simulink model "Control_Simulation"  (R2015a)
settings: Solver=ode45  StartTime=0.0  StopTime=15000  MaxStep=1  RelTol=1e-3
InitFcn:
  | m = 1.33;
  | L = 0.1;
  | Jxx = m*L^2/12;
  | Jyy = m*L^2/12;
  | Jzz = m*L^2/12;
  | J = diag([Jxx, Jyy, Jzz]);
  | omega0 = [1 1 1];
  | 
  | phi0=0;
  | theta0=0;
  | psi0=0;
  | 
  | R0_ECIF_2_B = eye(3);
values from neighbouring files (symbols this model uses):
  Earth = wgs84Ellipsoid    [TrovaSorvoloConAngoli.m]    (also in calculate_orbit.m)
undefined symbols (not defined in the file or in its folder): WGS84
libraries: aerolibtransform2 x2, aerolib6dof2 x1, aerolibgravity2 x1
settings Model: Creator=mehdi  LastModifiedBy=mehdi

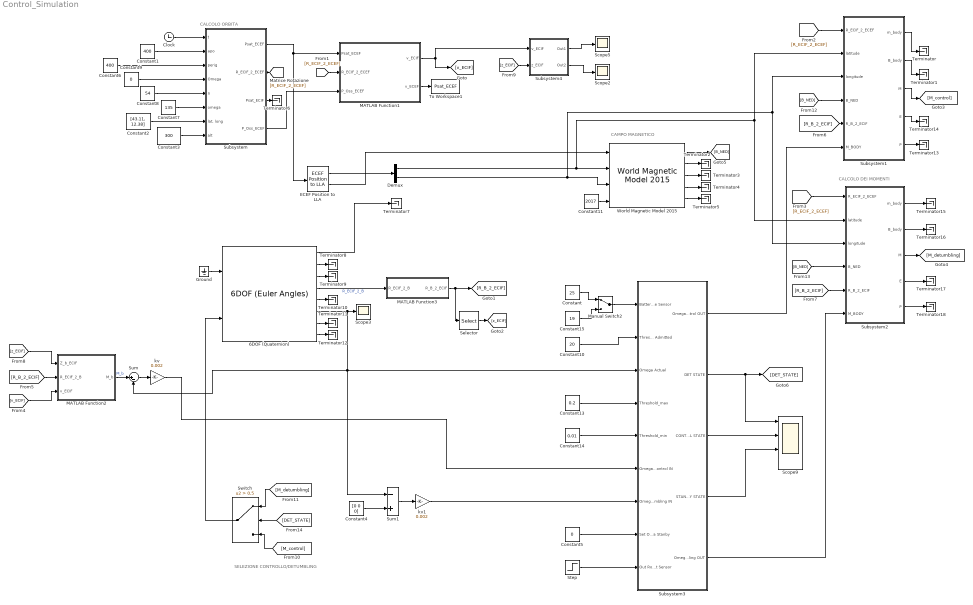
== system Control_Simulation ==
  note: SELEZIONE CONTROLLO/DETUMBLING
  note: CALCOLO DEI MOMENTI
  note: CAMPO MAGNETICO
  note: CALCOLO ORBITA
  6DOF (Quaternion) : aerolib6dof2/6DOF (Euler Angles)  units=Metric (MKS)  mtype=Fixed  rep=Quaternion  xme_0=[0 0 0]  Vm_0=[0 0 0]  eul_0=[0 0 0]  pm_0=omega0  mass_0=1.0  mass_e=0.5  mass_f=2.0  inertia=J  inertia_e=eye(3)  inertia_f=2*eye(3)  k_quat=1  vre_flag=on
  Clock : Clock
  Constant : Constant  Value=25
  Constant1 : Constant  Value=400
  Constant10 : Constant  Value=20
  Constant11 : Constant  Value=2017
  Constant13 : Constant  Value=0.2
  Constant14 : Constant  Value=0.01
  Constant15 : Constant  Value=19
  Constant2 : Constant  Value=[43.11, 12.38]
  Constant3 : Constant  Value=300
  Constant4 : Constant  Value=[0 0 0]
  Constant5 : Constant  Value=0
  Constant6 : Constant  Value=400
  Constant7 : Constant  Value=135
  Constant8 : Constant  Value=54
  Constant9 : Constant  Value=0
  Demux : Demux  Outputs=2
  ECEF Position to LLA : aerolibtransform2/ECEF Position to LLA  units=Metric (MKS)  ptype=Earth (WGS84)  F=1/298.257223563  R=6378137
  Ground : Ground
  MATLAB Function1 : MATLAB Function  TreatAsAtomicUnit=on
  MATLAB Function2 : MATLAB Function  TreatAsAtomicUnit=on
  MATLAB Function3 : MATLAB Function  TreatAsAtomicUnit=on
  Manual Switch2 : ManualSwitch
  Scope2 : Scope
      settings: YMin=0  YMax=14
  Scope3 : Scope
      settings: ShowLegends=on  YMin=-0.225  YMax=0.05  SaveName=v_ang
  Scope5 : Scope
      settings: YMin=-0.015  YMax=0.0175  SaveName=error_w
  Scope9 : Scope  NumInputPorts=4
      settings: TimeRange=1.404786680541292  YMin=-5~-5~-5~-5  YMax=5~5~5~5  SaveName=ScopeData8
  Selector : Selector  NumberOfDimensions=2  InputPortWidth=3  IndexOptions=Index vector (dialog),Index vector (dialog)  Indices=[1 2 3],3  OutputSizes=1,1
  Step : Step  SampleTime=0
  Subsystem : Subsystem
  Subsystem1 : Subsystem
  Subsystem2 : Subsystem
  Subsystem3 : Subsystem
  Subsystem4 : Subsystem
  Sum : Sum  Inputs=|+-
  Sum1 : Sum  Inputs=-+
  Switch : Switch  Criteria=u2 > Threshold  Threshold=0.5
  Terminator{,1..18} (19 alike) : Terminator
  To Workspace1 : ToWorkspace  VariableName=Psat_ECEF  SaveFormat=Structure With Time  SampleTime=-1
  World Magnetic Model 2015 : aerolibgravity2/World Magnetic Model 2015  units=Metric (MKS)  time_in=on  month=January  day=1  year=2015  action=Error  h_out=on  dec_out=on  inc_out=on  ti_out=on
  kv : Gain  Gain=0.002
  kv1 : Gain  Gain=0.002
  wires:
  MATLAB Function2/1(M_b) -> Sum/1  "M_b"
  6DOF (Quaternion)/4 -> MATLAB Function3/1(R_ECIF_2_B)  "R_ECIF_2_B"
  MATLAB Function3/1(R_B_2_ECIF) -> Selector/1, [R_B_2_ECIF]
  Sum/1 -> kv/1
  Clock/1 -> Subsystem/1(t)
  Constant1/1 -> Subsystem/2(apo)
  Constant6/1 -> Subsystem/3(perig)
  Constant9/1 -> Subsystem/4(Omega)
  Constant8/1 -> Subsystem/5(Ii)
  Constant7/1 -> Subsystem/6(omega)
  Constant2/1 -> Subsystem/7("lat, long")
  Constant3/1 -> Subsystem/8(alt)
  Subsystem/4(P_Oss_ECEF) -> MATLAB Function1/3(P_Oss_ECEF)
  Subsystem/1(Psat_ECEF) -> ECEF Position to LLA/1, MATLAB Function1/1(Psat_ECEF)
  ECEF Position to LLA/2 -> World Magnetic Model 2015/1
  Demux/1 -> World Magnetic Model 2015/2, Subsystem1/2(latitude), Subsystem2/2(latitude)
  Demux/2 -> Subsystem2/3(longitude), Subsystem1/3(longitude), World Magnetic Model 2015/3
  ECEF Position to LLA/1 -> Demux/1
  Subsystem1/2(B_body) -> Terminator1/1
  Constant11/1 -> World Magnetic Model 2015/4
  Subsystem1/1(m_body) -> Terminator/1
  MATLAB Function1/2(v_ECEF) -> To Workspace1/1
  World Magnetic Model 2015/2 -> Terminator2/1
  World Magnetic Model 2015/3 -> Terminator3/1
  World Magnetic Model 2015/4 -> Terminator4/1
  World Magnetic Model 2015/5 -> Terminator5/1
  Subsystem/3(Psat_ECIF) -> Terminator6/1
  6DOF (Quaternion)/1 -> Terminator7/1
  6DOF (Quaternion)/2 -> Terminator8/1
  6DOF (Quaternion)/3 -> Terminator9/1
  6DOF (Quaternion)/5 -> Terminator10/1
  6DOF (Quaternion)/7 -> Terminator11/1
  6DOF (Quaternion)/8 -> Terminator12/1
  Ground/1 -> 6DOF (Quaternion)/1
  6DOF (Quaternion)/6 -> Sum1/1, Subsystem3/3(Omega Actual), Sum/2, Scope3/1
  Constant4/1 -> Sum1/2
  Sum1/1 -> kv1/1
  Switch/1 -> 6DOF (Quaternion)/2
  Subsystem/2(R_ECIF_2_ECEF) -> [R_ECIF_2_ECEF]
  [R_ECIF_2_ECEF] -> MATLAB Function1/2(R_ECIF_2_ECEF)
  [R_ECIF_2_ECEF] -> Subsystem1/1(R_ECIF_2_ECEF)
  [R_ECIF_2_ECEF] -> Subsystem2/1(R_ECIF_2_ECEF)
  Constant10/1 -> Subsystem3/2(Threshold Admitted)
  Constant5/1 -> Subsystem3/8(Set Omega Stanby)
  Constant13/1 -> Subsystem3/4(Threshold_max)
  Constant14/1 -> Subsystem3/5(Threshold_min)
  Constant/1 -> Manual Switch2/1
  Constant15/1 -> Manual Switch2/2
  Manual Switch2/1 -> Subsystem3/1(Battery Charge Sensor)
  Subsystem3/2(DET STATE) -> [DET_STATE], Scope9/1
  Subsystem3/3(CONTROL STATE) -> Scope9/2
  Subsystem3/4(STANDBY STATE) -> Scope9/3
  Step/1 -> Subsystem3/9(Out Rocket Sensor)
  kv1/1 -> Subsystem3/7(Omega Dethumbling IN)
  kv/1 -> Subsystem3/6(Omega Control IN)
  Subsystem3/5(Omega Dethumbling OUT) -> Subsystem2/6(M_BODY)
  Subsystem3/1(Omega Control OUT) -> Subsystem1/6(M_BODY)
  Subsystem4/1(Out1) -> Scope5/1
  Subsystem4/2(Out2) -> Scope2/1
  Subsystem1/4(E) -> Terminator14/1
  Subsystem1/5("P ") -> Terminator13/1
  Subsystem2/1(m_body) -> Terminator15/1
  Subsystem2/2(B_body) -> Terminator16/1
  Subsystem2/4(E) -> Terminator17/1
  Subsystem2/5("P ") -> Terminator18/1
  MATLAB Function1/1(v_ECIF) -> Subsystem4/1(v_ECIF), [v_ECIF]
  [v_ECIF] -> MATLAB Function2/3(v_ECIF)
  [R_B_2_ECIF] -> MATLAB Function2/2(R_ECIF_2_B)
  [R_B_2_ECIF] -> Subsystem1/5(R_B_2_ECIF)
  [R_B_2_ECIF] -> Subsystem2/5(R_B_2_ECIF)
  Selector/1 -> [z_ECIF]
  [z_ECIF] -> MATLAB Function2/1(Z_b_ECIF)
  [z_ECIF] -> Subsystem4/2(z_ECIF)
  Subsystem1/3(M) -> [M_control]
  [M_control] -> Switch/3
  [M_detumbling] -> Switch/1
  Subsystem2/3(M) -> [M_detumbling]
  World Magnetic Model 2015/1 -> [B_NED]
  [B_NED] -> Subsystem1/4(B_NED)
  [B_NED] -> Subsystem2/4(B_NED)
  [DET_STATE] -> Switch/2

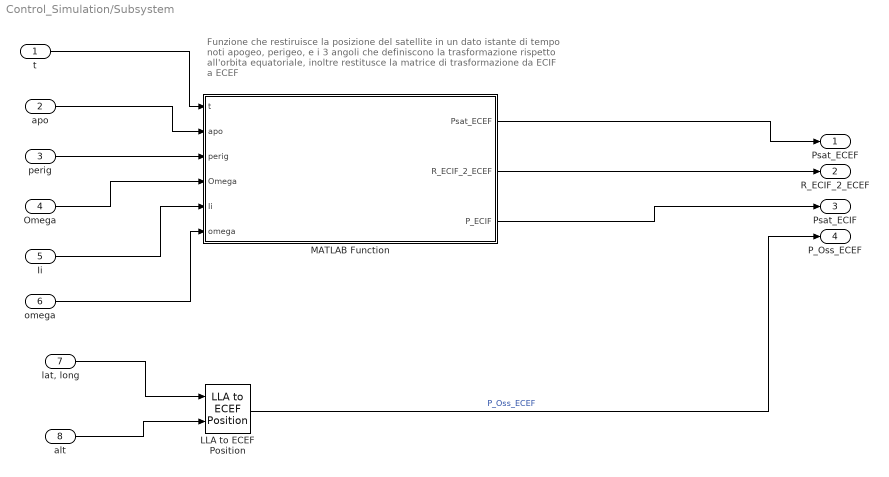
== system Control_Simulation/Subsystem ==
  note: Funzione che restiruisce la posizione del satellite in un dato
      | istante di tempo noti apogeo, perigeo, e i 3 angoli che definiscono
      | la trasformazione rispetto all'orbita equatoriale, inoltre
      | restitusce la matrice di trasformazione da ECIF a ECEF
  t : Inport
  apo : Inport  Port=2
  perig : Inport  Port=3
  Omega : Inport  Port=4
  Ii : Inport  Port=5
  omega : Inport  Port=6
  "lat, long" : Inport  Port=7
  alt : Inport  Port=8
  LLA to ECEF Position : aerolibtransform2/LLA to ECEF Position  units=Metric (MKS)  ptype=Earth (WGS84)  F=1/298.257223563  R=6378137
  MATLAB Function : MATLAB Function  TreatAsAtomicUnit=on
  Psat_ECEF : Outport
  R_ECIF_2_ECEF : Outport  Port=2
  Psat_ECIF : Outport  Port=3
  P_Oss_ECEF : Outport  Port=4
  wires:
  MATLAB Function/3(P_ECIF) -> Psat_ECIF/1
  t/1 -> MATLAB Function/1(t)
  apo/1 -> MATLAB Function/2(apo)
  perig/1 -> MATLAB Function/3(perig)
  omega/1 -> MATLAB Function/6(omega)
  Ii/1 -> MATLAB Function/5(Ii)
  Omega/1 -> MATLAB Function/4(Omega)
  alt/1 -> LLA to ECEF Position/2
  MATLAB Function/2(R_ECIF_2_ECEF) -> R_ECIF_2_ECEF/1
  LLA to ECEF Position/1 -> P_Oss_ECEF/1  "P_Oss_ECEF"
  "lat, long"/1 -> LLA to ECEF Position/1
  MATLAB Function/1(Psat_ECEF) -> Psat_ECEF/1

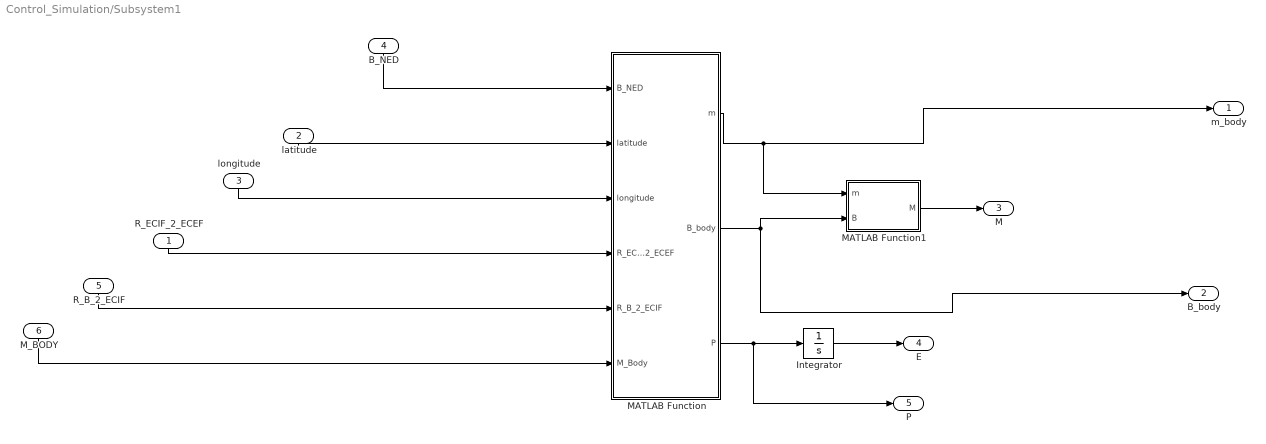
== system Control_Simulation/Subsystem1 ==
  R_ECIF_2_ECEF : Inport
  latitude : Inport  Port=2
  longitude : Inport  Port=3
  B_NED : Inport  Port=4
  R_B_2_ECIF : Inport  Port=5
  M_BODY : Inport  Port=6
  Integrator : Integrator
  MATLAB Function : MATLAB Function  TreatAsAtomicUnit=on
  MATLAB Function1 : MATLAB Function  TreatAsAtomicUnit=on
  m_body : Outport
  B_body : Outport  Port=2
  M : Outport  Port=3
  E : Outport  Port=4
  "P " : Outport  Port=5
  wires:
  B_NED/1 -> MATLAB Function/1(B_NED)
  R_B_2_ECIF/1 -> MATLAB Function/5(R_B_2_ECIF)
  longitude/1 -> MATLAB Function/3(longitude)
  R_ECIF_2_ECEF/1 -> MATLAB Function/4(R_ECIF_2_ECEF)
  latitude/1 -> MATLAB Function/2(latitude)
  MATLAB Function/1(m) -> MATLAB Function1/1(m), m_body/1
  M_BODY/1 -> MATLAB Function/6(M_Body)
  MATLAB Function/2(B_body) -> B_body/1, MATLAB Function1/2(B)
  MATLAB Function1/1(M) -> M/1
  MATLAB Function/3(P) -> "P "/1, Integrator/1
  Integrator/1 -> E/1

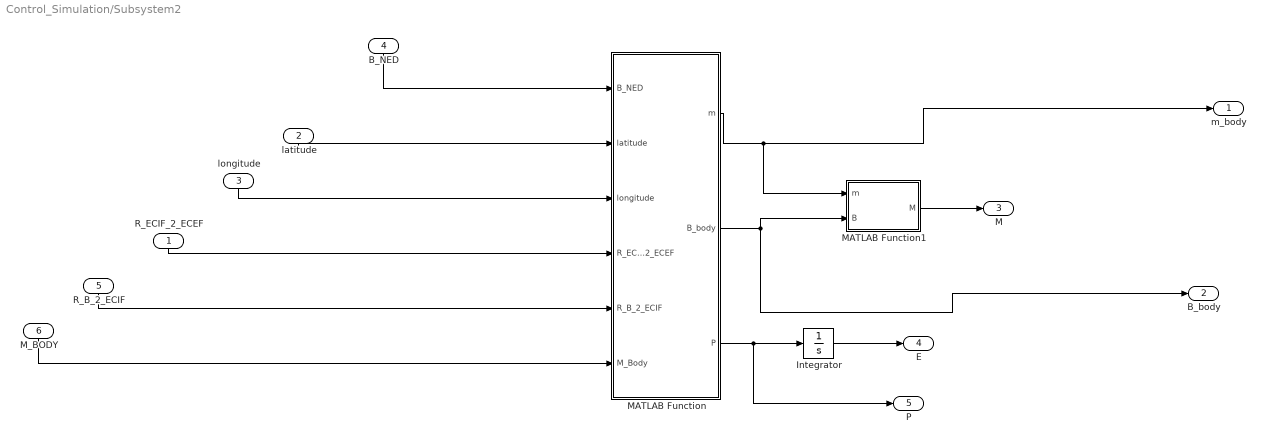
== system Control_Simulation/Subsystem2 ==
  R_ECIF_2_ECEF : Inport
  latitude : Inport  Port=2
  longitude : Inport  Port=3
  B_NED : Inport  Port=4
  R_B_2_ECIF : Inport  Port=5
  M_BODY : Inport  Port=6
  Integrator : Integrator
  MATLAB Function : MATLAB Function  TreatAsAtomicUnit=on
  MATLAB Function1 : MATLAB Function  TreatAsAtomicUnit=on
  m_body : Outport
  B_body : Outport  Port=2
  M : Outport  Port=3
  E : Outport  Port=4
  "P " : Outport  Port=5
  wires:
  B_NED/1 -> MATLAB Function/1(B_NED)
  R_B_2_ECIF/1 -> MATLAB Function/5(R_B_2_ECIF)
  longitude/1 -> MATLAB Function/3(longitude)
  R_ECIF_2_ECEF/1 -> MATLAB Function/4(R_ECIF_2_ECEF)
  latitude/1 -> MATLAB Function/2(latitude)
  MATLAB Function/1(m) -> MATLAB Function1/1(m), m_body/1
  M_BODY/1 -> MATLAB Function/6(M_Body)
  MATLAB Function/2(B_body) -> B_body/1, MATLAB Function1/2(B)
  MATLAB Function1/1(M) -> M/1
  MATLAB Function/3(P) -> "P "/1, Integrator/1
  Integrator/1 -> E/1

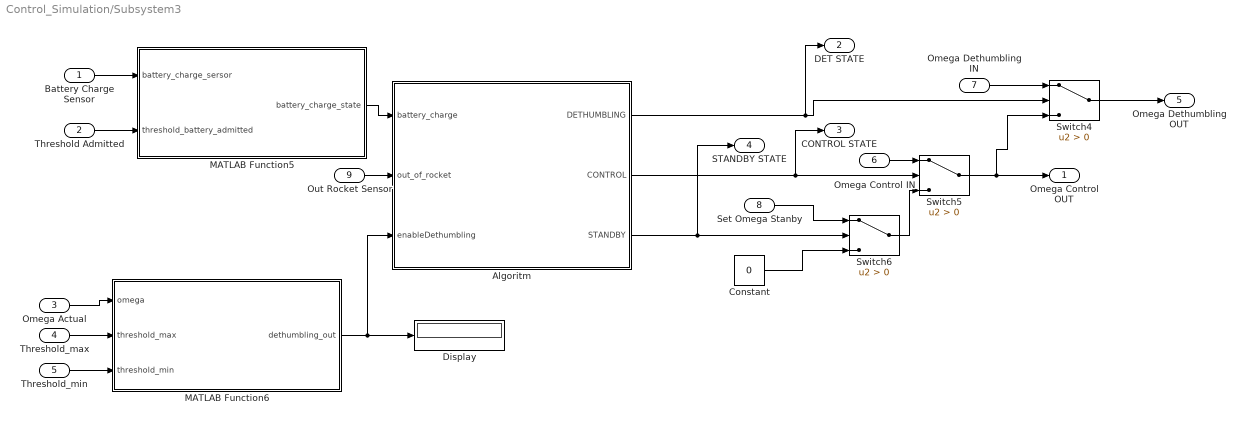
== system Control_Simulation/Subsystem3 ==
  Battery Charge Sensor : Inport
  Threshold Admitted : Inport  Port=2
  Omega Actual : Inport  Port=3
  Threshold_max : Inport  Port=4
  Threshold_min : Inport  Port=5
  Omega Control IN : Inport  Port=6
  Omega Dethumbling IN : Inport  Port=7
  Set Omega Stanby : Inport  Port=8
  Out Rocket Sensor : Inport  Port=9
  Algoritm : Stateflow chart  TreatAsAtomicUnit=on
  Constant : Constant  Value=0
  Display : Display
  MATLAB Function5 : MATLAB Function  TreatAsAtomicUnit=on
  MATLAB Function6 : MATLAB Function  TreatAsAtomicUnit=on
  Switch4 : Switch  Criteria=u2 > Threshold
  Switch5 : Switch  Criteria=u2 > Threshold
  Switch6 : Switch  Criteria=u2 > Threshold
  Omega Control OUT : Outport
  DET STATE : Outport  Port=2
  CONTROL STATE : Outport  Port=3
  STANDBY STATE : Outport  Port=4
  Omega Dethumbling OUT : Outport  Port=5
  wires:
  Threshold_max/1 -> MATLAB Function6/2(threshold_max)
  Omega Actual/1 -> MATLAB Function6/1(omega)
  Battery Charge Sensor/1 -> MATLAB Function5/1(battery_charge_sersor)
  Threshold Admitted/1 -> MATLAB Function5/2(threshold_battery_admitted)
  MATLAB Function5/1(battery_charge_state) -> Algoritm/1(battery_charge)
  MATLAB Function6/1(dethumbling_out) -> Algoritm/3(enableDethumbling), Display/1
  Algoritm/3(STANDBY) -> STANDBY STATE/1, Switch6/2
  Algoritm/2(CONTROL) -> CONTROL STATE/1, Switch5/2
  Algoritm/1(DETHUMBLING) -> DET STATE/1, Switch4/2
  Switch6/1 -> Switch5/3
  Switch5/1 -> Switch4/3, Omega Control OUT/1
  Switch4/1 -> Omega Dethumbling OUT/1
  Omega Control IN/1 -> Switch5/1
  Omega Dethumbling IN/1 -> Switch4/1
  Set Omega Stanby/1 -> Switch6/1
  Constant/1 -> Switch6/3
  Out Rocket Sensor/1 -> Algoritm/2(out_of_rocket)
  Threshold_min/1 -> MATLAB Function6/3(threshold_min)

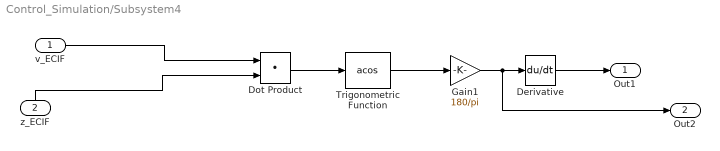
== system Control_Simulation/Subsystem4 ==
  v_ECIF : Inport
  z_ECIF : Inport  Port=2
  Derivative : Derivative
  Dot Product : DotProduct  InputSameDT=on  OutDataTypeStr=Inherit: Inherit via internal rule
  Gain1 : Gain  Gain=180/pi
  Trigonometric Function : Trigonometry  Operator=acos
  Out1 : Outport
  Out2 : Outport  Port=2
  wires:
  Dot Product/1 -> Trigonometric Function/1
  Trigonometric Function/1 -> Gain1/1
  Derivative/1 -> Out1/1
  Gain1/1 -> Out2/1, Derivative/1
  z_ECIF/1 -> Dot Product/2
  v_ECIF/1 -> Dot Product/1

== matlab function Control_Simulation/MATLAB Function1 ==
  data: Psat_ECEF input; R_ECIF_2_ECEF input; P_Oss_ECEF input; v_ECIF output; v_ECEF output
function [v_ECIF,v_ECEF] = fcn(Psat_ECEF, R_ECIF_2_ECEF, P_Oss_ECEF)

P_Os = P_Oss_ECEF - Psat_ECEF;
v_ECEF = P_Os/norm(P_Os);
v_ECIF = R_ECIF_2_ECEF*v_ECEF;

== matlab function Control_Simulation/Subsystem/MATLAB Function ==
  data: t input; Psat_ECEF output; apo input; perig input; Omega input; Ii input; omega input; R_ECIF_2_ECEF output; P_ECIF output
function [Psat_ECEF, R_ECIF_2_ECEF, P_ECIF] = orbita_riferimento(t,apo,perig,Omega,Ii,omega)

% Restituisce in coordinate ECEF la posizione del satellite in funzione
% dell'orbita desiderata, che viene calcolata con i parametri in ingresso:
% 
% IN:
%   t: tempo, in secondi
%   apo: apogeo dell'orbita
%   perig: perigeo dell'orbita
%   Omega: longitudine del nodo ascendente
%   Ii: inclinazione
%   omega: longitudine del perigeo
%
% OUT:
%   Psat_ECEF: vettore contenente la posizione del sattallite in coordinate
%   ECEF lungo l'orbita disegnata
%

R_Terra = 6371;

r_peri = (R_Terra+perig)*1000;
r_apo = (R_Terra+apo)*1000;
a = (r_apo+r_peri)/2;
e = (r_apo-r_peri)/(r_apo+r_peri);

Tterra = 86164.090530833; %% giorno siderale
omegaTerra = 2*pi/Tterra;
GM = 0.398601234780431e15;
T = 2*pi*a^1.5/sqrt(GM);

Omega = Omega*pi/180;
Ii = Ii*pi/180;
omega = omega*pi/180;

R1 = [cos(Omega),-sin(Omega),0;sin(Omega),cos(Omega),0;0,0,1];
R2 = [1,0,0;0,cos(Ii),-sin(Ii);0,sin(Ii),cos(Ii)];
R3 = [cos(omega),-sin(omega),0;sin(omega),cos(omega),0;0,0,1];
R = R1*R2*R3;

M=2*pi*t/T;
E1=M;
E=e*sin(E1)+M;

tol = 1e-6; % tolleranza a cui ritenere risolto l'espressione iterativa
while(abs(E-E1)>tol);
    E=E1;
    E1=e*sin(E)+M;
end

ra = (1-e*cos(E));
sv = sqrt(1-e^2)*sin(E)/ra;
cv = (cos(E)-e)/ra;
P0 = a*[ra*sv;ra*cv;0];
P_ECIF = R*P0;
theta = omegaTerra*t;
ct = cos(theta);
st = sin(theta);
R_ECIF_2_ECEF = [ct,-st,0; st,ct,0; 0,0,1]; 
Psat_ECEF = R_ECIF_2_ECEF'*P_ECIF;

omega_sat = 2*pi/T;
v_sat = omega_sat*Psat_ECEF;

== matlab function Control_Simulation/MATLAB Function3 ==
  data: R_ECIF_2_B input; R_B_2_ECIF output
function R_B_2_ECIF = fcn(R_ECIF_2_B)
%#codegen
R_B_2_ECIF = R_ECIF_2_B';

== matlab function Control_Simulation/Subsystem2/MATLAB Function ==
  data: B_NED input; m output; latitude input; longitude input; R_ECIF_2_ECEF input; R_B_2_ECIF input; M_Body input; B_body output; P output
function [m, B_body, P] = fcn(B_NED, latitude, longitude, R_ECIF_2_ECEF, R_B_2_ECIF, M_Body)
%#codegen
lambda = latitude;
theta = longitude;
sla=sin(lambda);
cla=cos(lambda);
sth=sin(theta);
cth=cos(theta);

%R_ECEF_2_NED = [-sin(lambda)*cos(theta), -sin(lambda)*sin(theta), cos(lambda);
%                -sin(theta), cos(theta), 0;
%                -cos(lambda)*cos(theta), -cos(lambda)*sin(theta), sin(lambda)];
R_ECEF_2_NED = [-sla*cth, -sla*sth, cla;
                -sth, cth, 0;
                -cla*cth, -cla*sth, sla];

            
R_B_2_NED = (R_B_2_ECIF)*(R_ECIF_2_ECEF)*(R_ECEF_2_NED);

B_body = R_B_2_NED*B_NED*(10^-9);

B_x = B_body(1);
B_y = B_body(2);
B_z = B_body(3);

M_x = M_Body(1);
M_y = M_Body(2);
M_z = M_Body(3);

%m_x = (M_y*B_x^2 - B_y*M_x*B_x + M_y*B_z^2 - B_y*M_z*B_z)/(B_x^2*B_z + B_y^2*B_z + B_z^3);
%m_y = -(M_x*B_y^2 - B_x*M_y*B_y + M_x*B_z^2 - B_x*M_z*B_z)/(B_x^2*B_z + B_y^2*B_z + B_z^3);
%m_z = 0;

m_x =  ((B_body(3)*M_Body(2)) - (B_body(2)*M_Body(3)));
m_y =  ((B_body(1)*M_Body(3)) - (B_body(3)*M_Body(1)));
m_z = -((B_body(1)*M_Body(2) - B_body(2)*M_Body(1)));

m = [m_x, m_y, m_z]/(norm(B_body)^2); 

% in questa sezione viene applicata la saturazione "manualemnte" in modo da
% non modificare la direzione. Altrimenti se si applica il saturatore
% vengono modiificate modificate le direzioni a causa dei ricalcoli che
% vengono fatto
m_max = 0.12;

k_x = abs(m(1)/m_max);
k_y = abs(m(2)/m_max);
k_z = abs(m(3)/m_max);

k = max([k_x, k_y, k_z]);

if k>1
    m = m/k;
end

P = m(1)^2 + m(2)^2 + m(3)^2;

== matlab function Control_Simulation/MATLAB Function2 ==
  data: Z_b_ECIF input; R_ECIF_2_B input; v_ECIF input; M_b output
function M_b = fcn(Z_b_ECIF, R_ECIF_2_B, v_ECIF)

k=0.05;
% in questa funzione definiamo il momento da applicare come il prodotto
% scalare tra i due assi da allineare (a meno del fattore di guadagno che 
% aggiusta le grandezze), infatti il prodotto scalare è quella funzione che
% "porta" il vettore Z_b_ECIF sul vettore v_ECIF, moltiplicando il tutto
% per la trasposta della matrice R_ECIF_2_B ottengo il risultato nelle
% coordinate Body.

M_b = (R_ECIF_2_B')*cross(Z_b_ECIF, v_ECIF)*k;

== matlab function Control_Simulation/Subsystem1/MATLAB Function ==
  data: B_NED input; m output; latitude input; longitude input; R_ECIF_2_ECEF input; R_B_2_ECIF input; M_Body input; B_body output; P output
function [m, B_body, P] = fcn(B_NED, latitude, longitude, R_ECIF_2_ECEF, R_B_2_ECIF, M_Body)
%#codegen
lambda = latitude;
theta = longitude;
sla=sin(lambda);
cla=cos(lambda);
sth=sin(theta);
cth=cos(theta);

%R_ECEF_2_NED = [-sin(lambda)*cos(theta), -sin(lambda)*sin(theta), cos(lambda);
%                -sin(theta), cos(theta), 0;
%                -cos(lambda)*cos(theta), -cos(lambda)*sin(theta), sin(lambda)];
R_ECEF_2_NED = [-sla*cth, -sla*sth, cla;
                -sth, cth, 0;
                -cla*cth, -cla*sth, sla];

            
R_B_2_NED = (R_B_2_ECIF)*(R_ECIF_2_ECEF)*(R_ECEF_2_NED);

B_body = R_B_2_NED*B_NED*(10^-9);

B_x = B_body(1);
B_y = B_body(2);
B_z = B_body(3);

M_x = M_Body(1);
M_y = M_Body(2);
M_z = M_Body(3);

%m_x = (M_y*B_x^2 - B_y*M_x*B_x + M_y*B_z^2 - B_y*M_z*B_z)/(B_x^2*B_z + B_y^2*B_z + B_z^3);
%m_y = -(M_x*B_y^2 - B_x*M_y*B_y + M_x*B_z^2 - B_x*M_z*B_z)/(B_x^2*B_z + B_y^2*B_z + B_z^3);
%m_z = 0;

m_x =  (B_body(3)*M_Body(2));
m_y = -(B_body(3)*M_Body(1));
m_z = -((B_body(1)*M_Body(2) - B_body(2)*M_Body(1)));

m = [m_x, m_y, m_z]/(norm(B_body)^2); 

% in questa sezione viene applicata la saturazione "manualemnte" in modo da
% non modificare la direzione. Altrimenti se si applica il saturatore
% vengono modiificate modificate le direzioni a causa dei ricalcoli che
% vengono fatto
m_max = 0.12;

k_x = abs(m(1)/m_max);
k_y = abs(m(2)/m_max);
k_z = abs(m(3)/m_max);

k = max([k_x, k_y, k_z]);

if k>1
    m = m/k;
end

P = m(1)^2 + m(2)^2 + m(3)^2;

== matlab function Control_Simulation/Subsystem1/MATLAB Function1 ==
  data: m input; M output; B input
function M = fcn(m, B)

M = -cross(m, B);

== matlab function Control_Simulation/Subsystem2/MATLAB Function1 ==
  data: m input; M output; B input
function M = fcn(m, B)

M = -cross(m, B);

== stateflow chart Control_Simulation/Subsystem3/Algoritm ==
  state STANDBY
    entry:
    CONTROL=0;
    DETHUMBLING=0;
    STANDBY=1;
  state DETHUMBLING
    entry:
    CONTROL=0;
    DETHUMBLING=1;
    STANDBY=0;
  state CONTROL
    entry:
    CONTROL=1;
    DETHUMBLING=0;
    STANDBY=0;
  CONTROL -> STANDBY [order 2] : [battery_charge==0 && out_of_rocket==1]
  (default) -> STANDBY
  STANDBY -> DETHUMBLING [order 2] : [out_of_rocket==1 && battery_charge==1 && enableDethumbling==1 && after(5, sec)]
  DETHUMBLING -> CONTROL [order 1] : [enableDethumbling==0 && after(15, sec)]
  DETHUMBLING -> STANDBY [order 2] : [battery_charge==0 && out_of_rocket==1]
  CONTROL -> DETHUMBLING [order 1] : [enableDethumbling==1 && after(15, sec)]
  STANDBY -> CONTROL [order 1] : [out_of_rocket==1 && battery_charge==1 && enableDethumbling==1 && after(5, sec)]
  data: battery_charge input; out_of_rocket input; DETHUMBLING output; CONTROL output; STANDBY output; enableDethumbling input

== matlab function Control_Simulation/Subsystem3/MATLAB Function5 ==
  data: battery_charge_sersor input; battery_charge_state output; threshold_battery_admitted input
function battery_charge_state = fcn(battery_charge_sersor,threshold_battery_admitted)
    battery_charge_state=0;
%     under this threshold the system going to standby
    if(battery_charge_sersor>threshold_battery_admitted)
            battery_charge_state=1;
        else
            battery_charge_state=0;
    end
end

== matlab function Control_Simulation/Subsystem3/MATLAB Function6 ==
  data: omega input; dethumbling_out output; threshold_max input; threshold_min input
function dethumbling_out = fcn(omega,threshold_max,threshold_min)
% upper this threshold enable a request for turn on dethumbling
    persistent request_dethumbling_state
    if (isempty(request_dethumbling_state))
        request_dethumbling_state = 1;
    end
    if(abs(omega(1))>threshold_max|abs(omega(2))>threshold_max|abs(omega(3))>threshold_max)
            request_dethumbling_state=1;
    end
    if(abs(omega(1))<threshold_min & abs(omega(2))<threshold_min & abs(omega(3))<threshold_min)
            request_dethumbling_state=0;
    end
    
    dethumbling_out=request_dethumbling_state;
end
